simulink model "dinamicaDoRoboLista3"  (R2022a)
settings: Solver=VariableStepAuto  StartTime=0.0  StopTime=10.0  RelTol=1e-3
values from neighbouring files (symbols this model uses):
  K = 1    [scriptLista3.m]
  r = 1/50    (= 0.02)    [scriptLista3.m]
settings Model: Creator=vfton  LastModifiedBy=vfton

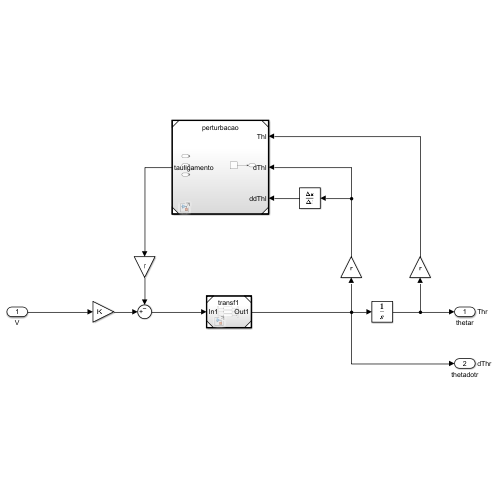
[thumbnail: Simulink's stored preview of the top-level diagram]
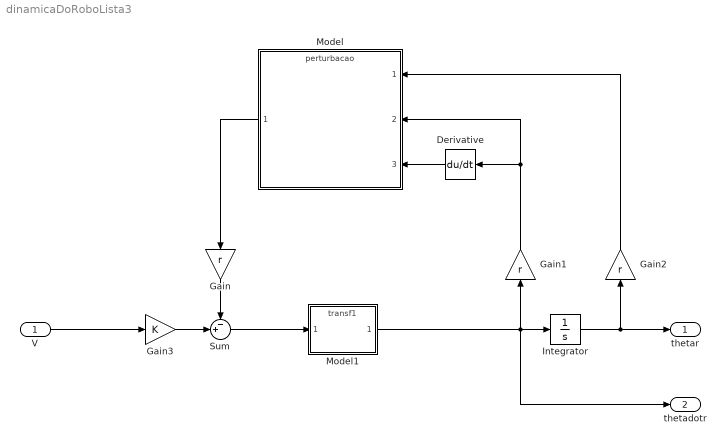
== system dinamicaDoRoboLista3 ==
  V : Inport  PortDimensions=3
  Derivative : Derivative
  Gain : Gain  Gain=r
  Gain1 : Gain  Gain=r
  Gain2 : Gain  Gain=r
  Gain3 : Gain  Gain=K
  Integrator : Integrator
  Model : ModelReference  ModelNameDialog=perturbacao.slx  SimulationMode=Normal  ModelReferenceVersion=1.6
  Model1 : ModelReference  ModelNameDialog=transf1.slx  SimulationMode=Normal  ModelReferenceVersion=1.1
  Sum : Sum  Inputs=-+|
  thetar : Outport  SignalName=Thr  PortDimensions=3
  thetadotr : Outport  Port=2  SignalName=dThr  PortDimensions=3
  wires:
  Gain3/1 -> Sum/2
  Integrator/1 -> thetar/1, Gain2/1
  Gain1/1 -> Model/2, Derivative/1
  Model1/1 -> thetadotr/1, Integrator/1, Gain1/1
  Gain/1 -> Sum/1
  Sum/1 -> Model1/1
  Derivative/1 -> Model/3
  Gain2/1 -> Model/1
  Model/1 -> Gain/1
  V/1 -> Gain3/1
